simulink model "math_sqrt_test"  (Simulink 8.7)
settings: Solver=VariableStepDiscrete  StartTime=0.0  StopTime=10.0  RelTol=1e-3
undefined symbols (not defined in the file or in its folder): Newton, Raphson
settings Model: Creator=arnaud  LastModifiedBy=hamza
settings DataIOCC: SaveFormat=Structure  SignalLoggingSaveFormat=ModelDataLogs
settings OptimizationCC: ExpressionDepthLimit=2147483647
settings DebuggingCC: SolverPrmCheckMsg=warning  FcnCallInpInsideContextMsg=UseLocalSettings  StateNameClashWarn=warning
settings GRTTargetCC: CombineOutputUpdateFcns=off  GRTInterface=on
settings ConfigComp: CovSFcnEnable=off

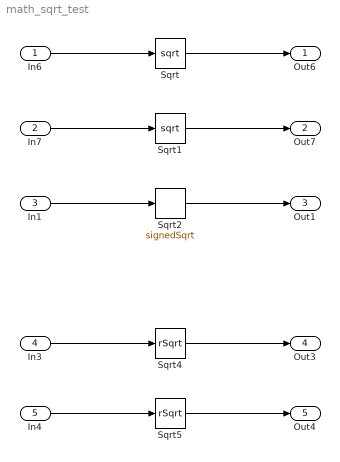
== system math_sqrt_test ==
  In6 : Inport  OutDataTypeStr=uint32
  In7 : Inport  Port=2  OutDataTypeStr=uint32
  In1 : Inport  Port=3
  In3 : Inport  Port=4  OutDataTypeStr=double
  In4 : Inport  Port=5  OutDataTypeStr=uint32
  Sqrt : Sqrt  SaturateOnIntegerOverflow=on
  Sqrt1 : Sqrt  SaturateOnIntegerOverflow=on
  Sqrt2 : Sqrt  Operator=signedSqrt  SaturateOnIntegerOverflow=on
  Sqrt4 : Sqrt  Operator=rSqrt  SaturateOnIntegerOverflow=on
  Sqrt5 : Sqrt  Operator=rSqrt  AlgorithmType=Newton-Raphson  SaturateOnIntegerOverflow=on
  Out6 : Outport
  Out7 : Outport  Port=2
  Out1 : Outport  Port=3
  Out3 : Outport  Port=4
  Out4 : Outport  Port=5
  wires:
  In6/1 -> Sqrt/1
  Sqrt/1 -> Out6/1
  In7/1 -> Sqrt1/1
  Sqrt1/1 -> Out7/1
  In1/1 -> Sqrt2/1
  Sqrt2/1 -> Out1/1
  In3/1 -> Sqrt4/1
  Sqrt4/1 -> Out3/1
  In4/1 -> Sqrt5/1
  Sqrt5/1 -> Out4/1
